simulink model "E4_Desequilibrio"  (R2018a)
settings: Solver=VariableStepAuto  StartTime=0.0  StopTime=0.5  RelTol=1e-3
libraries: powerlib x37, powerlib_meascontrol x24
settings Model: Creator=Rafael Pavan  LastModifiedBy=Rafael Pavan

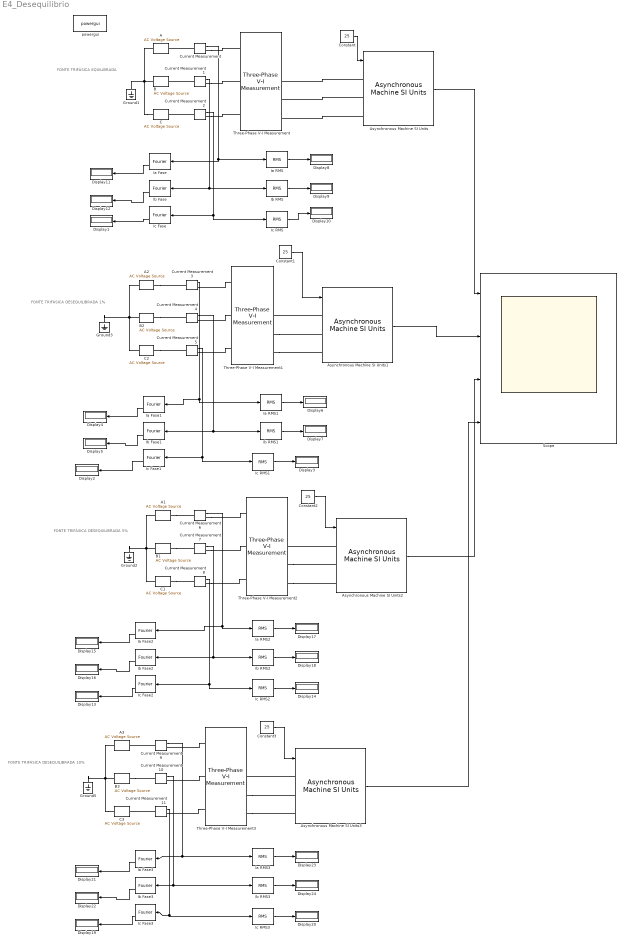
== system E4_Desequilibrio ==
  note: FONTE TRIFÁSICA EQUILIBRADA
  note: FONTE TRIFÁSICA DESEQUILIBRADA 1%
  note: FONTE TRIFÁSICA DESEQUILIBRADA 5%
  note: FONTE TRIFÁSICA DESEQUILIBRADA 10%
  A : powerlib/Electrical Sources/AC Voltage Source  Amplitude=179.605  Phase=0  Frequency=60  SampleTime=0  Measurements=None  BusType=PV  Pref=100e4  Qref=0  Qmin=-inf  Qmax=+inf
  A1 : powerlib/Electrical Sources/AC Voltage Source  Amplitude=179.605  Phase=0  Frequency=60  SampleTime=0  Measurements=None  BusType=PV  Pref=100e4  Qref=0  Qmin=-inf  Qmax=+inf
  A2 : powerlib/Electrical Sources/AC Voltage Source  Amplitude=179.6051224  Phase=0  Frequency=60  SampleTime=0  Measurements=None  BusType=PV  Pref=100e4  Qref=0  Qmin=-inf  Qmax=+inf
  A3 : powerlib/Electrical Sources/AC Voltage Source  Amplitude=179.6051224  Phase=0  Frequency=60  SampleTime=0  Measurements=None  BusType=PV  Pref=100e4  Qref=0  Qmin=-inf  Qmax=+inf
  Asynchronous Machine SI Units{,1..3} (4 alike) : powerlib/Machines/Asynchronous Machine SI Units  RotorType=Squirrel-cage  PresetModel=No  MechanicalLoad=Torque Tm  ShowDetailedParameters=on  ReferenceFrame=Rotor  Units=SI  MeasurementBus=off  NominalParameters=[38105 220 60]  Stator=[0.5968 0.0003495]  Rotor=[0.6258 0.005473]  Cage1=[0.4155 0.002066]  Cage2=[0.4168 0.0003495]  Lm=0.0354  Mechanical=[0.05 0.005879 3]  PolePairs=2  InitialConditions=[0.03 0 0 0 0 0 0 0]  SimulateSaturation=off  Saturation=[14.03593122, 27.81365428, 53.79336849, 72.68890987, 97.98006896, 148.6815601, 215.7428561, 302.9841135, 428.7778367 ; 230, 322, 414, 460, 506, 552, 598, 644, 690]  LoadFlowParameters=1492000  TsPowergui=0  TsBlock=-1  IterativeModel=Trapezoidal non iterative  IterativeDiscreteModel=Trapezoidal non iterative  Pmec=29150
  B : powerlib/Electrical Sources/AC Voltage Source  Amplitude=179.605  Phase=-120  Frequency=60  SampleTime=0  Measurements=None  BusType=PV  Pref=100e4  Qref=0  Qmin=-inf  Qmax=+inf
  B1 : powerlib/Electrical Sources/AC Voltage Source  Amplitude=193.46  Phase=-120  Frequency=60  SampleTime=0  Measurements=None  BusType=PV  Pref=100e4  Qref=0  Qmin=-inf  Qmax=+inf
  B2 : powerlib/Electrical Sources/AC Voltage Source  Amplitude=181.019336  Phase=-120  Frequency=60  SampleTime=0  Measurements=None  BusType=PV  Pref=100e4  Qref=0  Qmin=-inf  Qmax=+inf
  B3 : powerlib/Electrical Sources/AC Voltage Source  Amplitude=207.3237082  Phase=-120  Frequency=60  SampleTime=0  Measurements=None  BusType=PV  Pref=100e4  Qref=0  Qmin=-inf  Qmax=+inf
  C : powerlib/Electrical Sources/AC Voltage Source  Amplitude=179.605  Phase=120  Frequency=60  SampleTime=0  Measurements=None  BusType=PV  Pref=100e4  Qref=0  Qmin=-inf  Qmax=+inf
  C1 : powerlib/Electrical Sources/AC Voltage Source  Amplitude=162.63  Phase=120  Frequency=60  SampleTime=0  Measurements=None  BusType=PV  Pref=100e4  Qref=0  Qmin=-inf  Qmax=+inf
  C2 : powerlib/Electrical Sources/AC Voltage Source  Amplitude=175.07  Phase=120  Frequency=60  SampleTime=0  Measurements=None  BusType=PV  Pref=100e4  Qref=0  Qmin=-inf  Qmax=+inf
  C3 : powerlib/Electrical Sources/AC Voltage Source  Amplitude=145.6639969  Phase=120  Frequency=60  SampleTime=0  Measurements=None  BusType=PV  Pref=100e4  Qref=0  Qmin=-inf  Qmax=+inf
  Constant{,1..3} (4 alike) : Constant  Value=25
  Current Measurement{,1..11} (12 alike) : powerlib/Measurements/Current Measurement  PhasorSimulation=off  OutputType=Complex  PSBequivalent=0
  Display{1..24} (24 alike) : Display
  Ground{1..3,5} (4 alike) : powerlib/Elements/Ground  LConnTagsString=a
  Ia Fase{,1..3} (4 alike) : powerlib_meascontrol/Measurements/Fourier  Freq=60  n=1  InInit=[0, 0]  Ts=0
      settings: SourceProductName=Simscape Power Systems
  Ia RMS{,1..3} (4 alike) : powerlib_meascontrol/Measurements/RMS  TrueRMS=on  Freq=60  RMSInit=120  Ts=0
  Ib Fase{,1..3} (4 alike) : powerlib_meascontrol/Measurements/Fourier  Freq=60  n=1  InInit=[0, 0]  Ts=0
      settings: SourceProductName=Simscape Power Systems
  Ib RMS{,1..3} (4 alike) : powerlib_meascontrol/Measurements/RMS  TrueRMS=on  Freq=60  RMSInit=120  Ts=0
  Ic Fase{,1..3} (4 alike) : powerlib_meascontrol/Measurements/Fourier  Freq=60  n=1  InInit=[0, 0]  Ts=0
      settings: SourceProductName=Simscape Power Systems
  Ic RMS{,1..3} (4 alike) : powerlib_meascontrol/Measurements/RMS  TrueRMS=on  Freq=60  RMSInit=120  Ts=0
  Scope : Scope  NumInputPorts=4
  Three-Phase V-I Measurement{,1..3} (4 alike) : powerlib/Measurements/Three-Phase V-I Measurement  VoltageMeasurement=phase-to-ground  SetLabelV=off  LabelV=Vabc  Vpu=off  VpuLL=off  CurrentMeasurement=yes  SetLabelI=off  LabelI=Iabc  Ipu=off  Pbase=100e6  Vbase=500e3  OutputType=Complex  PhasorSimulation=off  PSBequivalent=0
  powergui : powerlib/powergui  Priority=1  SimulationMode=Continuous  SampleTime=50e-6  frequency=60  Iterations=50  frequencyindice=60  Pbase=100e6  ErrMax=1e-4  UnitsV=kV  UnitsW=MW  buscounter=0  FunctionMessages=on  echomessages=off  EnableUseOfTLC=off  CurrentSourceSwitches=off  DisableSnubberDevices=off  DisableRonSwitches=off  DisableVfSwitches=off  DisplayEquations=off  SolverType=Tustin/Backward Euler (TBE)  Interpol=off  ExternalGateDelay=off  methode=off  Ts=100  x0status=blocks  SPID=on  SwTol=0  HookPort=off  RestoreLinks=warning  ResistiveCurrentMeasurement=off  Frange=[0:2:500]  Ylog=off  Xlog=on  ShowGrid=off  save=off  variable=ZData  structure=0  ZoomFFT=off  StartTime=0.0  cycles=1  DisplayStyle=1  fundamental=60  FreqAxis=off  MaxFrequency=1000  frequencyindicesteady=1  RmsSteady=2  display=off
  wires:
  Asynchronous Machine SI Units/1 -> Scope/1
  Constant/1 -> Asynchronous Machine SI Units/1
  Constant1/1 -> Asynchronous Machine SI Units1/1
  Asynchronous Machine SI Units1/1 -> Scope/2
  Constant2/1 -> Asynchronous Machine SI Units2/1
  Asynchronous Machine SI Units2/1 -> Scope/3
  Constant3/1 -> Asynchronous Machine SI Units3/1
  Asynchronous Machine SI Units3/1 -> Scope/4
  Ib RMS/1 -> Display9/1
  Ia Fase/2 -> Display11/1
  Ic RMS/1 -> Display10/1
  Ia RMS/1 -> Display8/1
  Ib Fase/2 -> Display12/1
  Ic Fase/2 -> Display1/1
  Ic Fase1/2 -> Display2/1
  Ia RMS1/1 -> Display6/1
  Ib RMS1/1 -> Display7/1
  Ib Fase1/2 -> Display5/1
  Ic RMS1/1 -> Display3/1
  Ia Fase1/2 -> Display4/1
  Ic Fase2/2 -> Display13/1
  Ia RMS2/1 -> Display17/1
  Ib RMS2/1 -> Display18/1
  Ib Fase2/2 -> Display16/1
  Ic RMS2/1 -> Display14/1
  Ia Fase2/2 -> Display15/1
  Ic Fase3/2 -> Display19/1
  Ia RMS3/1 -> Display23/1
  Ib RMS3/1 -> Display24/1
  Ib Fase3/2 -> Display22/1
  Ic RMS3/1 -> Display20/1
  Ia Fase3/2 -> Display21/1
  Current Measurement2/1 -> Ic Fase/1, Ic RMS/1
  Current Measurement1/1 -> Ib Fase/1, Ib RMS/1
  Current Measurement/1 -> Ia Fase/1, Ia RMS/1
  Current Measurement5/1 -> Ic RMS1/1, Ic Fase1/1
  Current Measurement4/1 -> Ib RMS1/1, Ib Fase1/1
  Current Measurement3/1 -> Ia Fase1/1, Ia RMS1/1
  Current Measurement6/1 -> Ia Fase2/1, Ia RMS2/1
  Current Measurement7/1 -> Ib Fase2/1, Ib RMS2/1
  Current Measurement8/1 -> Ic Fase2/1, Ic RMS2/1
  Current Measurement9/1 -> Ia Fase3/1, Ia RMS3/1
  Current Measurement10/1 -> Ib Fase3/1, Ib RMS3/1
  Current Measurement11/1 -> Ic Fase3/1, Ic RMS3/1
  connections:
  C/LConn1 -- B/LConn1 -- Ground1/LConn1 -- A/LConn1
  B1/LConn1 -- Ground2/LConn1 -- A1/LConn1 -- C1/LConn1
  A2/LConn1 -- Ground3/LConn1 -- C2/LConn1 -- B2/LConn1
  C3/LConn1 -- B3/LConn1 -- Ground5/LConn1 -- A3/LConn1
  Asynchronous Machine SI Units/LConn2 -- Three-Phase V-I Measurement/RConn2
  Asynchronous Machine SI Units/LConn1 -- Three-Phase V-I Measurement/RConn1
  Asynchronous Machine SI Units/LConn3 -- Three-Phase V-I Measurement/RConn3
  Asynchronous Machine SI Units1/LConn1 -- Three-Phase V-I Measurement1/RConn1
  Three-Phase V-I Measurement1/RConn2 -- Asynchronous Machine SI Units1/LConn2
  Three-Phase V-I Measurement1/RConn3 -- Asynchronous Machine SI Units1/LConn3
  Three-Phase V-I Measurement2/RConn2 -- Asynchronous Machine SI Units2/LConn2
  Three-Phase V-I Measurement2/RConn3 -- Asynchronous Machine SI Units2/LConn3
  Asynchronous Machine SI Units2/LConn1 -- Three-Phase V-I Measurement2/RConn1
  Asynchronous Machine SI Units3/LConn1 -- Three-Phase V-I Measurement3/RConn1
  Three-Phase V-I Measurement3/RConn3 -- Asynchronous Machine SI Units3/LConn3
  Three-Phase V-I Measurement3/RConn2 -- Asynchronous Machine SI Units3/LConn2
  Current Measurement/LConn1 -- A/RConn1
  Current Measurement/RConn1 -- Three-Phase V-I Measurement/LConn1
  Current Measurement1/LConn1 -- B/RConn1
  Current Measurement1/RConn1 -- Three-Phase V-I Measurement/LConn2
  Current Measurement2/LConn1 -- C/RConn1
  Current Measurement2/RConn1 -- Three-Phase V-I Measurement/LConn3
  B2/RConn1 -- Current Measurement4/LConn1
  Three-Phase V-I Measurement1/LConn1 -- Current Measurement3/RConn1
  A2/RConn1 -- Current Measurement3/LConn1
  Three-Phase V-I Measurement1/LConn2 -- Current Measurement4/RConn1
  C2/RConn1 -- Current Measurement5/LConn1
  Three-Phase V-I Measurement1/LConn3 -- Current Measurement5/RConn1
  B1/RConn1 -- Current Measurement7/LConn1
  Current Measurement6/RConn1 -- Three-Phase V-I Measurement2/LConn1
  A1/RConn1 -- Current Measurement6/LConn1
  Current Measurement7/RConn1 -- Three-Phase V-I Measurement2/LConn2
  C1/RConn1 -- Current Measurement8/LConn1
  Current Measurement8/RConn1 -- Three-Phase V-I Measurement2/LConn3
  Three-Phase V-I Measurement3/LConn2 -- Current Measurement10/RConn1
  Three-Phase V-I Measurement3/LConn3 -- Current Measurement11/RConn1
  Three-Phase V-I Measurement3/LConn1 -- Current Measurement9/RConn1
  Current Measurement9/LConn1 -- A3/RConn1
  B3/RConn1 -- Current Measurement10/LConn1
  Current Measurement11/LConn1 -- C3/RConn1
